simulink model "LAB_sim"  (R2022b)
settings: Solver=VariableStepAuto  StartTime=0.0  StopTime=1  RelTol=1e-3
values from neighbouring files (symbols this model uses):
  k = par(1)    [LAB_1_grafiks_angle.m]    (also in LAB_1_grafiks_omega.m; lab_1.m)
  Tm = par(2)    [LAB_1_grafiks_angle.m]    (also in LAB_1_grafiks_omega.m; lab_1.m)
  U_pr = voltages(i)    [LAB_1_grafiks_angle.m]    (also in LAB_1_grafiks_omega.m; lab_1.m)
settings Model: Creator=ppotr  LastModifiedBy=ppotr

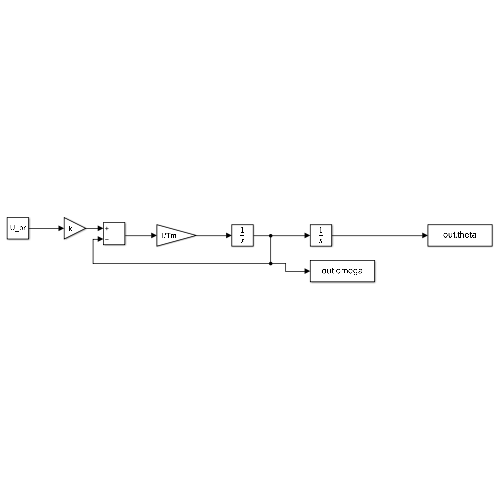
[thumbnail: Simulink's stored preview of the top-level diagram]
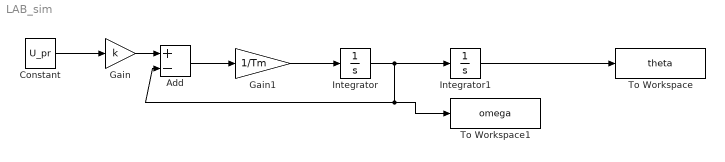
== system LAB_sim ==
  Add : Sum  Inputs=+-
  Constant : Constant  Value=U_pr
  Gain : Gain  Gain=k
  Gain1 : Gain  Gain=1/Tm
  Integrator : Integrator
  Integrator1 : Integrator
  To Workspace : ToWorkspace  VariableName=theta  SaveFormat=Timeseries  SampleTime=-1
  To Workspace1 : ToWorkspace  VariableName=omega  SaveFormat=Timeseries  SampleTime=-1
  wires:
  Constant/1 -> Gain/1
  Gain/1 -> Add/1
  Gain1/1 -> Integrator/1
  Add/1 -> Gain1/1
  Integrator1/1 -> To Workspace/1
  Integrator/1 -> Integrator1/1, To Workspace1/1, Add/2
